simulink model "motor_mixer"  (R2016a)
settings: Solver=VariableStepAuto  StartTime=0.0  StopTime=10.0  RelTol=1e-3
settings Model: Creator=GusBus  LastModifiedBy=GusBus
settings GRTTargetCC: GeneratePreprocessorConditionals=Use local settings

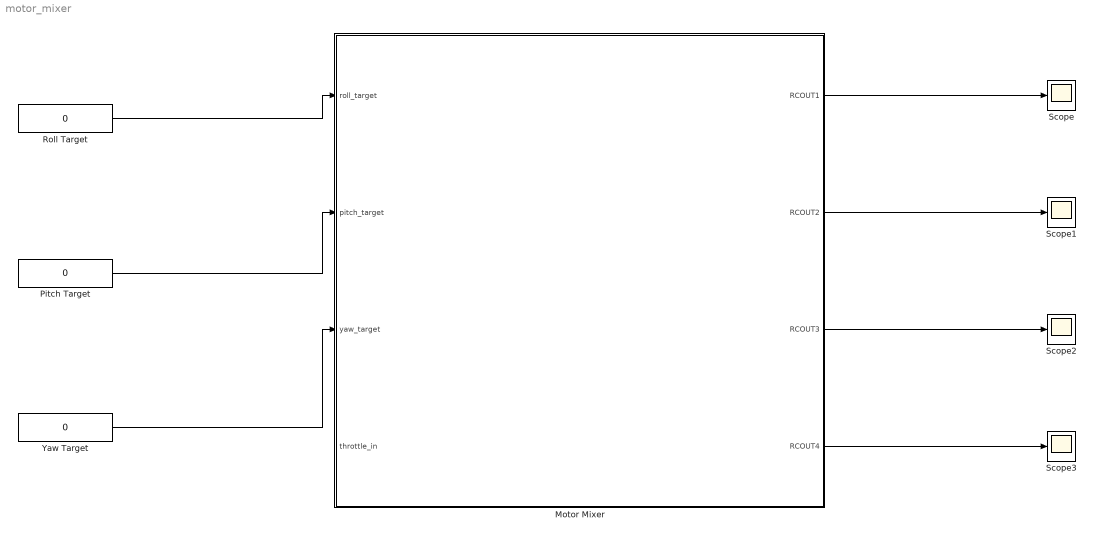
== system motor_mixer ==
  Motor Mixer : MATLAB Function  TreatAsAtomicUnit=on
  Pitch Target : Constant  Value=0
  Roll Target : Constant  Value=0
  Scope{,1..3} (4 alike) : Scope
  Yaw Target : Constant  Value=0
  wires:
  Roll Target/1 -> Motor Mixer/1(roll_target)
  Pitch Target/1 -> Motor Mixer/2(pitch_target)
  Yaw Target/1 -> Motor Mixer/3(yaw_target)
  Motor Mixer/1(RCOUT1) -> Scope/1
  Motor Mixer/2(RCOUT2) -> Scope1/1
  Motor Mixer/3(RCOUT3) -> Scope2/1
  Motor Mixer/4(RCOUT4) -> Scope3/1

== matlab function motor_mixer/Motor Mixer ==
  data: roll_target input; RCOUT1 output; pitch_target input; yaw_target input; RCOUT2 output; RCOUT3 output; RCOUT4 output; throttle_in input
function [RCOUT1, RCOUT2, RCOUT3, RCOUT4 ]  = motor_mixer( roll_target, pitch_target, yaw_target,throttle_in)
%% Motor Mixer

%
%   Matlab Implementation of the ArduPilot Motor Mixer
%   Outputs Motor Commands based on required rate targets
%
%
load('global.mat')



    % Update throttle filter
    update_throttle_filter(throttle_in);

    % Update battery resistance
    % update_battery_resistance();
                                                                            %For the model, we will always assume we have maximum lift
    % Calc filtered battery voltage and lift_max
    % update_lift_max_from_batt_voltage();

    % Run spool logic
    % output_logic();
    
    % Calculate thrust
    output_armed_stabilizing(roll_target, pitch_target, yaw_target);

    % Apply any thrust compensation for the frame
    % thrust_compensation();  %used for tilt rotors and tilt wings
    
    % Convert rpy_thrust values to pwm
    RCOUT1 = pwm_min + (pwm_max-pwm_min)*(spin_min + (spin_max-spin_min)*thrust_rpyt_out(1));
    RCOUT2 = pwm_min + (pwm_max-pwm_min)*(spin_min + (spin_max-spin_min)*thrust_rpyt_out(2));
    RCOUT3 = pwm_min + (pwm_max-pwm_min)*(spin_min + (spin_max-spin_min)*thrust_rpyt_out(3));
    RCOUT4 = pwm_min + (pwm_max-pwm_min)*(spin_min + (spin_max-spin_min)*thrust_rpyt_out(4));
    

end
